simulink model "SlidingMode_HW3_ClassicSMC"  (R2021a)
settings: Solver=VariableStepAuto  StartTime=0.0  StopTime=10.0  RelTol=1e-3
settings Model: Creator=kiankhaneghahi  LastModifiedBy=kiankhaneghahi
settings SolverCC: ZeroCrossAlgorithm=Adaptive
settings DebuggingCC: IgnoredZcDiagnostic=none

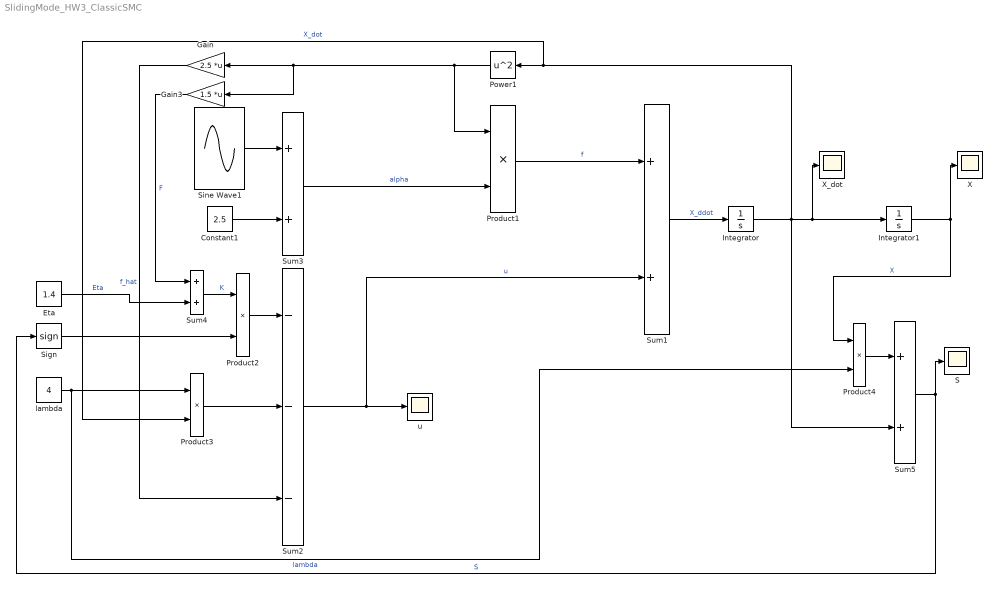
== system SlidingMode_HW3_ClassicSMC ==
  Constant1 : Constant  Value=2.5
  Eta : Constant  Value=1.4
  Gain : Gain  Gain=2.5  Multiplication=Matrix(K*u)
  Gain3 : Gain  Gain=1.5  Multiplication=Matrix(K*u)
  Integrator : Integrator  InitialCondition=1
  Integrator1 : Integrator  InitialCondition=2
  Power1 : Math  Operator=square  SaturateOnIntegerOverflow=on
  Product{1..4} (4 alike) : Product
  S : Scope
  Sign : Signum
  Sine Wave1 : Sin  Amplitude=1.5  SampleTime=0
  Sum{1,3..5} (4 alike) : Sum
  Sum2 : Sum  Inputs=---
  X : Scope
  X_dot : Scope
  lambda : Constant  Value=4
  u : Scope
  wires:
  Sum3/1 -> Product1/2  "alpha"
  Constant1/1 -> Sum3/2
  Gain/1 -> Sum2/3  "f_hat"
  Sum2/1 -> Sum1/2, u/1  "u"
  Integrator1/1 -> Product4/1, X/1  "X"
  Product1/1 -> Sum1/1  "f"
  Integrator/1 -> Sum5/2, Power1/1, Product3/2, X_dot/1, Integrator1/1  "X_dot"
  Product3/1 -> Sum2/2
  Sine Wave1/1 -> Sum3/1
  Sum1/1 -> Integrator/1  "X_ddot"
  Power1/1 -> Gain3/1, Gain/1, Product1/1
  Gain3/1 -> Sum4/1  "F"
  Sum4/1 -> Product2/1  "K"
  Eta/1 -> Sum4/2  "Eta"
  lambda/1 -> Product4/2, Product3/1  "lambda"
  Product2/1 -> Sum2/1
  Product4/1 -> Sum5/1
  Sum5/1 -> S/1, Sign/1  "S"
  Sign/1 -> Product2/2
